simulink library "firstOrdTrnsThm_ul"  (R2018b)
settings: Solver=VariableStepAuto  StartTime=0.0  StopTime=10.0  RelTol=1e-3
libraries: vrlib x1
settings Model: Creator=mcobb  LastModifiedBy=mcobb

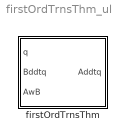
== system firstOrdTrnsThm_ul ==
  firstOrdTrnsThm : Subsystem

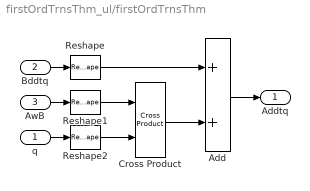
== system firstOrdTrnsThm_ul/firstOrdTrnsThm ==
  q : Inport  PortDimensions=3
  Bddtq : Inport  Port=2  PortDimensions=3
  AwB : Inport  Port=3  PortDimensions=3
  Add : Sum
  Cross Product : vrlib/Utilities/Cross Product
      settings: SourceProductBaseCode=VR
  Reshape : Reshape  OutputDimensionality=Column vector (2-D)
  Reshape1 : Reshape  OutputDimensionality=Column vector (2-D)
  Reshape2 : Reshape  OutputDimensionality=Column vector (2-D)
  Addtq : Outport  PortDimensions=3
  wires:
  Bddtq/1 -> Reshape/1
  Cross Product/1 -> Add/2
  AwB/1 -> Reshape1/1
  q/1 -> Reshape2/1
  Add/1 -> Addtq/1
  Reshape/1 -> Add/1
  Reshape1/1 -> Cross Product/1
  Reshape2/1 -> Cross Product/2
